simulink model "MdXX_RspChk"  (R2018b)
settings: Solver=FixedStepDiscrete  StartTime=0.0  StopTime=10.0  FixedStep=0.01  RelTol=1e-3
libraries: OutRspChkLib x20
(part 2 of 2)

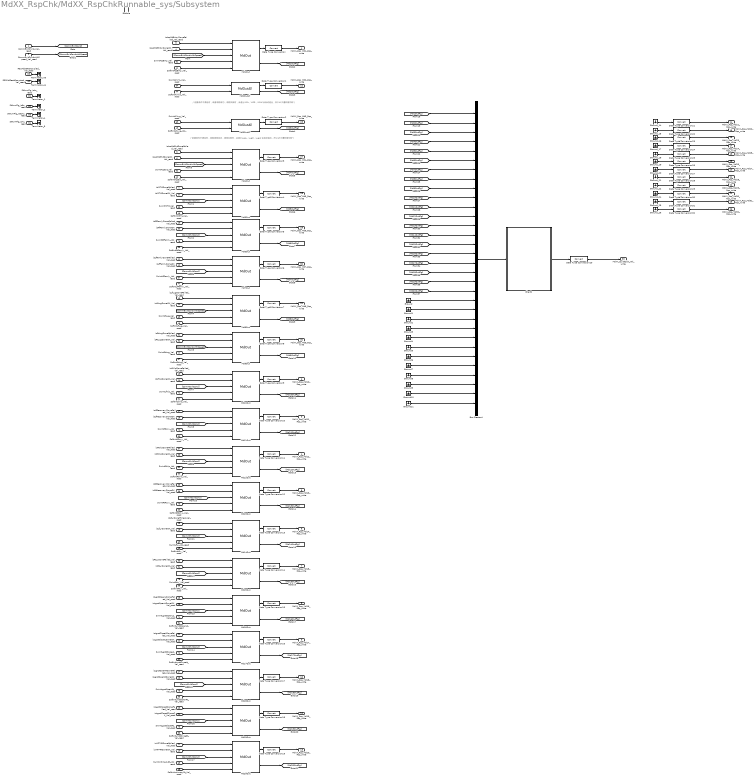
== system MdXX_RspChk/MdXX_RspChkRunnable_sys/Subsystem ==
  note: /*前提条件不满足时，或者调用成功，调用失败时，会退出LugL，LugR，LugAll会自动退出，所以All只看软硬中断*/
  note: /*前提条件不满足时，或者调用成功，调用失败时，会退出VIPL，VIPR，VIPAll会自动退出，所以All只看软硬中断*/
  CommExitCond_Val_read : Inport
  CommExitCondwithSpeed_Val_read : Inport  Port=2
  isAcsMdEntryDoneFailed_Val_read : Inport  Port=3
  isAcsMdEntryDoneOK_Val_read : Inport  Port=4
  isAcsMdExtDoneFailed_Val_read : Inport  Port=5
  isAcsMdExtDoneOK_Val_read : Inport  Port=6
  isINTMDoneFailed_Val_read : Inport  Port=7
  isINTMDoneOK_Val_read : Inport  Port=8
  isINTMRDoneFailed_Val_read : Inport  Port=9
  isINTMRDoneOK_Val_read : Inport  Port=10
  isLfFamlyDoneFailed_Val_read : Inport  Port=11
  isLfFamlyDoneOK_Val_read : Inport  Port=12
  isLfLugDoneFailed_Val_read : Inport  Port=13
  isLfLugDoneOK_Val_read : Inport  Port=14
  isLfLyDoneFailed_Val_read : Inport  Port=15
  isLfLyDoneOK_Val_read : Inport  Port=16
  isLfRecoveryDoneFailed_Val_read : Inport  Port=17
  isLfRecoveryDoneOK_Val_read : Inport  Port=18
  isLfVipDoneFailed_Val_read : Inport  Port=19
  isLfVipDoneOK_Val_read : Inport  Port=20
  isLgrstCloseLDoneFailed_Val_read : Inport  Port=21
  isLgrstCloseLDoneOK_Val_read : Inport  Port=22
  isLgrstCloseRDoneFailed_Val_read : Inport  Port=23
  isLgrstCloseRDoneOK_Val_read : Inport  Port=24
  isLgrstOpenLDoneFailed_Val_read : Inport  Port=25
  isLgrstOpenLDoneOK_Val_read : Inport  Port=26
  isLgrstOpenRDoneFailed_Val_read : Inport  Port=27
  isLgrstOpenRDoneOK_Val_read : Inport  Port=28
  isRfFamlyDoneFailed_Val_read : Inport  Port=29
  isRfFamlyDoneOK_Val_read : Inport  Port=30
  isRtLugDoneFailed_Val_read : Inport  Port=31
  isRtLugDoneOK_Val_read : Inport  Port=32
  isRtLyDoneFailed_Val_read : Inport  Port=33
  isRtLyDoneOK_Val_read : Inport  Port=34
  isRtRecoveryDoneFailed_Val_read : Inport  Port=35
  isRtRecoveryDoneOK_Val_read : Inport  Port=36
  isRtVipDoneFailed_Val_read : Inport  Port=37
  isRtVipDoneOK_Val_read : Inport  Port=38
  R3LMdSeatOccupied_Val_read : Inport  Port=39
  R3RMdSeatOccupied_Val_read : Inport  Port=40
  SoftIntAcsEnty_Val_read : Inport  Port=41
  SoftIntAcsExt_Val_read : Inport  Port=42
  SoftIntAllLug_Val_read : Inport  Port=43
  SoftIntAllVip_Val_read : Inport  Port=44
  SoftIntIntimacyRt_Val_read : Inport  Port=45
  SoftIntINTM_Val_read : Inport  Port=46
  SoftIntLfFamly_Val_read : Inport  Port=47
  SoftIntLfLug_Val_read : Inport  Port=48
  SoftIntLfLy_Val_read : Inport  Port=49
  SoftIntLfRcvy_Val_read : Inport  Port=50
  SoftIntLfVip_Val_read : Inport  Port=51
  SoftIntLgrstCloseLt_Val_read : Inport  Port=52
  SoftIntLgrstCloseRt_Val_read : Inport  Port=53
  SoftIntLgrstOpenLt_Val_read : Inport  Port=54
  SoftIntLgrstOpenRt_Val_read : Inport  Port=55
  SoftIntRtFamly_Val_read : Inport  Port=56
  SoftIntRtLug_Val_read : Inport  Port=57
  SoftIntRtLy_Val_read : Inport  Port=58
  SoftIntRtRcvy_Val_read : Inport  Port=59
  SoftIntRtVip_Val_read : Inport  Port=60
  SwIntAcsEnty_Val_read : Inport  Port=61
  SwIntAcsExt_Val_read : Inport  Port=62
  SwIntAllLug_Val_read : Inport  Port=63
  SwIntAllVip_Val_read : Inport  Port=64
  SwIntIntimacyRt_Val_read : Inport  Port=65
  SwIntINTM_Val_read : Inport  Port=66
  SwIntLfFamly_Val_read : Inport  Port=67
  SwIntLfLug_Val_read : Inport  Port=68
  SwIntLfLy_Val_read : Inport  Port=69
  SwIntLfRcvy_Val_read : Inport  Port=70
  SwIntLfVip_Val_read : Inport  Port=71
  SwIntLgrstCloseLt_Val_read : Inport  Port=72
  SwIntLgrstCloseRt_Val_read : Inport  Port=73
  SwIntLgrstOpenLt_Val_read : Inport  Port=74
  SwIntLgrstOpenRt_Val_read : Inport  Port=75
  SwIntRtFamly_Val_read : Inport  Port=76
  SwIntRtLug_Val_read : Inport  Port=77
  SwIntRtLy_Val_read : Inport  Port=78
  SwIntRtRcvy_Val_read : Inport  Port=79
  SwIntRtVip_Val_read : Inport  Port=80
  StNumFlg_Is4s_read : Inport  Port=81
  StNumFlg_Is6s_read : Inport  Port=82
  StNumFlg_Is6s7s_read : Inport  Port=83
  StNumFlg_Is7s_read : Inport  Port=84
  Enable : EnablePort
  Bus Creator4 : BusCreator  Inputs=32
  Chart2 : Stateflow chart  TreatAsAtomicUnit=on
  Data Type Conversion{,1..32} (33 alike) : DataTypeConversion
  Ground{,1..11} (12 alike) : Ground
  Ground_{14..22,24..26} (12 alike) : Ground
  Md10Out : OutRspChkLib/MdOut  SystemSampleTime=-1
  Md11Out : OutRspChkLib/MdOut  SystemSampleTime=-1
  Md12Out : OutRspChkLib/MdOut  SystemSampleTime=-1
  Md13Out : OutRspChkLib/MdOut  SystemSampleTime=-1
  Md14Out : OutRspChkLib/MdOut  SystemSampleTime=-1
  Md15Out : OutRspChkLib/MdOut  SystemSampleTime=-1
  Md16Out : OutRspChkLib/MdOut  SystemSampleTime=-1
  Md17Out : OutRspChkLib/MdOut  SystemSampleTime=-1
  Md18Out : OutRspChkLib/MdOut  SystemSampleTime=-1
  Md19Out : OutRspChkLib/MdOut  SystemSampleTime=-1
  Md1Out : OutRspChkLib/MdOut  SystemSampleTime=-1
  Md20Out : OutRspChkLib/MdOut  SystemSampleTime=-1
  Md2OutAll : OutRspChkLib/MdOutAll  SystemSampleTime=-1
  Md3OutAll : OutRspChkLib/MdOutAll  SystemSampleTime=-1
  Md4Out : OutRspChkLib/MdOut  SystemSampleTime=-1
  Md5Out : OutRspChkLib/MdOut  SystemSampleTime=-1
  Md6Out : OutRspChkLib/MdOut  SystemSampleTime=-1
  Md7Out : OutRspChkLib/MdOut  SystemSampleTime=-1
  Md8Out : OutRspChkLib/MdOut  SystemSampleTime=-1
  Md9Out : OutRspChkLib/MdOut  SystemSampleTime=-1
  Terminator_{1..2,4..5,43..44} (6 alike) : Terminator
  MdXX_Rsp_Md1_Rsp_write : Outport
  MdXX_Rsp_Md10_Rsp_write : Outport  Port=2
  MdXX_Rsp_Md11_Rsp_write : Outport  Port=3
  MdXX_Rsp_Md12_Rsp_write : Outport  Port=4
  MdXX_Rsp_Md13_Rsp_write : Outport  Port=5
  MdXX_Rsp_Md14_Rsp_write : Outport  Port=6
  MdXX_Rsp_Md15_Rsp_write : Outport  Port=7
  MdXX_Rsp_Md16_Rsp_write : Outport  Port=8
  MdXX_Rsp_Md17_Rsp_write : Outport  Port=9
  MdXX_Rsp_Md18_Rsp_write : Outport  Port=10
  MdXX_Rsp_Md19_Rsp_write : Outport  Port=11
  MdXX_Rsp_Md2_Rsp_write : Outport  Port=12
  MdXX_Rsp_Md20_Rsp_write : Outport  Port=13
  MdXX_Rsp_Md21_Rsp_write : Outport  Port=14
  MdXX_Rsp_Md22_Rsp_write : Outport  Port=15
  MdXX_Rsp_Md23_Rsp_write : Outport  Port=16
  MdXX_Rsp_Md24_Rsp_write : Outport  Port=17
  MdXX_Rsp_Md25_Rsp_write : Outport  Port=18
  MdXX_Rsp_Md26_Rsp_write : Outport  Port=19
  MdXX_Rsp_Md27_Rsp_write : Outport  Port=20
  MdXX_Rsp_Md28_Rsp_write : Outport  Port=21
  MdXX_Rsp_Md29_Rsp_write : Outport  Port=22
  MdXX_Rsp_Md3_Rsp_write : Outport  Port=23
  MdXX_Rsp_Md30_Rsp_write : Outport  Port=24
  MdXX_Rsp_Md31_Rsp_write : Outport  Port=25
  MdXX_Rsp_Md32_Rsp_write : Outport  Port=26
  MdXX_Rsp_Md4_Rsp_write : Outport  Port=27
  MdXX_Rsp_Md5_Rsp_write : Outport  Port=28
  MdXX_Rsp_Md6_Rsp_write : Outport  Port=29
  MdXX_Rsp_Md7_Rsp_write : Outport  Port=30
  MdXX_Rsp_Md8_Rsp_write : Outport  Port=31
  MdXX_Rsp_Md9_Rsp_write : Outport  Port=32
  MdXX_Quit32bit_Val_write : Outport  Port=33
  wires:
  isLfVipDoneFailed_Val_read/1 -> Md10Out/1
  Md1Out/1 -> Data Type Conversion/1
  Ground_18/1 -> Data Type Conversion25/1
  isLgrstOpenLDoneFailed_Val_read/1 -> Md16Out/1
  R3LMdSeatOccupied_Val_read/1 -> Terminator_43/1
  Ground_14/1 -> Data Type Conversion21/1
  SoftIntLgrstCloseRt_Val_read/1 -> Md19Out/5
  SwIntIntimacyRt_Val_read/1 -> Md20Out/4
  isLfFamlyDoneFailed_Val_read/1 -> Md7Out/1
  Ground_19/1 -> Data Type Conversion26/1
  Ground_24/1 -> Data Type Conversion30/1
  isRtVipDoneFailed_Val_read/1 -> Md12Out/1
  Ground_17/1 -> Data Type Conversion24/1
  Ground_20/1 -> Data Type Conversion27/1
  Ground_21/1 -> Data Type Conversion28/1
  isINTMDoneOK_Val_read/1 -> Md5Out/2
  isRfFamlyDoneOK_Val_read/1 -> Md6Out/2
  isLfLugDoneFailed_Val_read/1 -> Md8Out/1
  R3RMdSeatOccupied_Val_read/1 -> Terminator_44/1
  Ground_26/1 -> Data Type Conversion32/1
  isLgrstOpenLDoneOK_Val_read/1 -> Md16Out/2
  Ground_25/1 -> Data Type Conversion31/1
  isRtLugDoneOK_Val_read/1 -> Md9Out/2
  isRtLyDoneOK_Val_read/1 -> Md15Out/2
  isLfFamlyDoneOK_Val_read/1 -> Md7Out/2
  isLgrstOpenRDoneFailed_Val_read/1 -> Md18Out/1
  SoftIntLgrstOpenRt_Val_read/1 -> Md18Out/5
  isLfVipDoneOK_Val_read/1 -> Md10Out/2
  isRtVipDoneOK_Val_read/1 -> Md12Out/2
  CommExitCond_Val_read/1 -> [CommExitCond]
  isRtLyDoneFailed_Val_read/1 -> Md15Out/1
  isRfFamlyDoneFailed_Val_read/1 -> Md6Out/1
  isINTMDoneFailed_Val_read/1 -> Md5Out/1
  Ground_22/1 -> Data Type Conversion29/1
  isLgrstOpenRDoneOK_Val_read/1 -> Md18Out/2
  isINTMRDoneFailed_Val_read/1 -> Md20Out/1
  Ground_16/1 -> Data Type Conversion23/1
  Ground_15/1 -> Data Type Conversion22/1
  CommExitCondwithSpeed_Val_read/1 -> [CommExitCondwithSpeed]
  isLfRecoveryDoneOK_Val_read/1 -> Md11Out/2
  isLfRecoveryDoneFailed_Val_read/1 -> Md11Out/1
  isINTMRDoneOK_Val_read/1 -> Md20Out/2
  isLfLugDoneOK_Val_read/1 -> Md8Out/2
  isRtLugDoneFailed_Val_read/1 -> Md9Out/1
  SwIntAcsEnty_Val_read/1 -> Md1Out/4
  SoftIntAcsEnty_Val_read/1 -> Md1Out/5
  [CommExitCondwithSpeed] -> Md1Out/3
  isAcsMdEntryDoneFailed_Val_read/1 -> Md1Out/1
  isAcsMdEntryDoneOK_Val_read/1 -> Md1Out/2
  Md1Out/2 -> [Md1OutFlg]
  Md3OutAll/1 -> Data Type Conversion2/1
  Md2OutAll/1 -> Data Type Conversion1/1
  Md4Out/1 -> Data Type Conversion3/1
  Md5Out/1 -> Data Type Conversion4/1
  Md6Out/1 -> Data Type Conversion5/1
  Md7Out/1 -> Data Type Conversion6/1
  Md8Out/1 -> Data Type Conversion7/1
  Md9Out/1 -> Data Type Conversion8/1
  Md10Out/1 -> Data Type Conversion9/1
  Md11Out/1 -> Data Type Conversion10/1
  Md12Out/1 -> Data Type Conversion11/1
  Md13Out/1 -> Data Type Conversion12/1
  Md14Out/1 -> Data Type Conversion13/1
  Md15Out/1 -> Data Type Conversion14/1
  Md16Out/1 -> Data Type Conversion15/1
  Md17Out/1 -> Data Type Conversion16/1
  Md18Out/1 -> Data Type Conversion17/1
  Md19Out/1 -> Data Type Conversion18/1
  Md20Out/1 -> Data Type Conversion19/1
  Md2OutAll/2 -> [Md2OutFlg]
  Md3OutAll/2 -> [Md3OutFlg]
  Md4Out/2 -> [Md4OutFlg]
  Md5Out/2 -> [Md5OutFlg]
  Md6Out/2 -> [Md6OutFlg]
  Md7Out/2 -> [Md7OutFlg]
  Md8Out/2 -> [Md8OutFlg]
  Md9Out/2 -> [Md9OutFlg]
  Md10Out/2 -> [Md10OutFlg]
  Md11Out/2 -> [Md11OutFlg]
  Md12Out/2 -> [Md12OutFlg]
  Md13Out/2 -> [Md13OutFlg]
  Md14Out/2 -> [Md14OutFlg]
  Md15Out/2 -> [Md15OutFlg]
  Md16Out/2 -> [Md16OutFlg]
  Md17Out/2 -> [Md17OutFlg]
  Md18Out/2 -> [Md18OutFlg]
  Md19Out/2 -> [Md19OutFlg]
  Md20Out/2 -> [Md20OutFlg]
  isAcsMdExtDoneFailed_Val_read/1 -> Md4Out/1
  isAcsMdExtDoneOK_Val_read/1 -> Md4Out/2
  isRtRecoveryDoneFailed_Val_read/1 -> Md13Out/1
  isRtRecoveryDoneOK_Val_read/1 -> Md13Out/2
  isLfLyDoneFailed_Val_read/1 -> Md14Out/1
  isLfLyDoneOK_Val_read/1 -> Md14Out/2
  isLgrstCloseLDoneFailed_Val_read/1 -> Md17Out/1
  isLgrstCloseLDoneOK_Val_read/1 -> Md17Out/2
  isLgrstCloseRDoneFailed_Val_read/1 -> Md19Out/1
  isLgrstCloseRDoneOK_Val_read/1 -> Md19Out/2
  [CommExitCondwithSpeed] -> Md4Out/3
  [CommExitCondwithSpeed] -> Md8Out/3
  [CommExitCondwithSpeed] -> Md9Out/3
  [CommExitCond] -> Md5Out/3
  [CommExitCond] -> Md6Out/3
  [CommExitCond] -> Md7Out/3
  [CommExitCond] -> Md10Out/3
  [CommExitCond] -> Md11Out/3
  [CommExitCond] -> Md12Out/3
  [CommExitCond] -> Md13Out/3
  [CommExitCond] -> Md14Out/3
  [CommExitCond] -> Md15Out/3
  [CommExitCond] -> Md16Out/3
  [CommExitCond] -> Md17Out/3
  [CommExitCond] -> Md18Out/3
  [CommExitCond] -> Md19Out/3
  [CommExitCond] -> Md20Out/3
  SwIntLgrstCloseRt_Val_read/1 -> Md19Out/4
  SwIntLgrstOpenRt_Val_read/1 -> Md18Out/4
  SwIntLgrstOpenLt_Val_read/1 -> Md16Out/4
  SwIntLgrstCloseLt_Val_read/1 -> Md17Out/4
  SwIntRtLy_Val_read/1 -> Md15Out/4
  SwIntLfLy_Val_read/1 -> Md14Out/4
  SwIntRtRcvy_Val_read/1 -> Md13Out/4
  SwIntRtVip_Val_read/1 -> Md12Out/4
  SwIntLfRcvy_Val_read/1 -> Md11Out/4
  SwIntLfVip_Val_read/1 -> Md10Out/4
  SwIntLfLug_Val_read/1 -> Md8Out/4
  SwIntLfFamly_Val_read/1 -> Md7Out/4
  SwIntRtFamly_Val_read/1 -> Md6Out/4
  SwIntINTM_Val_read/1 -> Md5Out/4
  SoftIntAllLug_Val_read/1 -> Md3OutAll/2
  SoftIntAllVip_Val_read/1 -> Md2OutAll/2
  SoftIntINTM_Val_read/1 -> Md5Out/5
  SoftIntAcsExt_Val_read/1 -> Md4Out/5
  SwIntAllLug_Val_read/1 -> Md3OutAll/1
  SwIntAllVip_Val_read/1 -> Md2OutAll/1
  SwIntAcsExt_Val_read/1 -> Md4Out/4
  SoftIntLfFamly_Val_read/1 -> Md7Out/5
  SoftIntRtFamly_Val_read/1 -> Md6Out/5
  SwIntRtLug_Val_read/1 -> Md9Out/4
  SoftIntLfVip_Val_read/1 -> Md10Out/5
  SoftIntLfRcvy_Val_read/1 -> Md11Out/5
  SoftIntRtVip_Val_read/1 -> Md12Out/5
  SoftIntRtRcvy_Val_read/1 -> Md13Out/5
  SoftIntLfLy_Val_read/1 -> Md14Out/5
  SoftIntRtLy_Val_read/1 -> Md15Out/5
  SoftIntLgrstCloseLt_Val_read/1 -> Md17Out/5
  SoftIntRtLug_Val_read/1 -> Md9Out/5
  SoftIntLfLug_Val_read/1 -> Md8Out/5
  SoftIntIntimacyRt_Val_read/1 -> Md20Out/5
  Chart2/1(Data32Bit) -> Data Type Conversion20/1
  Bus Creator4/1 -> Chart2/1(DataArray)  "MdQuitFlg"
  [Md1OutFlg] -> Bus Creator4/1
  [Md2OutFlg] -> Bus Creator4/2
  [Md3OutFlg] -> Bus Creator4/3
  [Md4OutFlg] -> Bus Creator4/4
  [Md5OutFlg] -> Bus Creator4/5
  [Md6OutFlg] -> Bus Creator4/6
  [Md7OutFlg] -> Bus Creator4/7
  [Md8OutFlg] -> Bus Creator4/8
  [Md9OutFlg] -> Bus Creator4/9
  [Md10OutFlg] -> Bus Creator4/10
  [Md11OutFlg] -> Bus Creator4/11
  [Md12OutFlg] -> Bus Creator4/12
  [Md13OutFlg] -> Bus Creator4/13
  [Md14OutFlg] -> Bus Creator4/14
  [Md15OutFlg] -> Bus Creator4/15
  [Md16OutFlg] -> Bus Creator4/16
  [Md17OutFlg] -> Bus Creator4/17
  [Md18OutFlg] -> Bus Creator4/18
  [Md19OutFlg] -> Bus Creator4/19
  [Md20OutFlg] -> Bus Creator4/20
  Ground/1 -> Bus Creator4/21
  Ground1/1 -> Bus Creator4/22
  Ground2/1 -> Bus Creator4/23
  Ground3/1 -> Bus Creator4/24
  Ground4/1 -> Bus Creator4/25
  Ground5/1 -> Bus Creator4/26
  Ground6/1 -> Bus Creator4/27
  Ground7/1 -> Bus Creator4/28
  Ground8/1 -> Bus Creator4/29
  Ground9/1 -> Bus Creator4/30
  Ground10/1 -> Bus Creator4/31
  Ground11/1 -> Bus Creator4/32
  Data Type Conversion/1 -> MdXX_Rsp_Md1_Rsp_write/1
  Data Type Conversion1/1 -> MdXX_Rsp_Md2_Rsp_write/1
  Data Type Conversion2/1 -> MdXX_Rsp_Md3_Rsp_write/1
  Data Type Conversion3/1 -> MdXX_Rsp_Md4_Rsp_write/1
  Data Type Conversion4/1 -> MdXX_Rsp_Md5_Rsp_write/1
  Data Type Conversion5/1 -> MdXX_Rsp_Md6_Rsp_write/1
  Data Type Conversion6/1 -> MdXX_Rsp_Md7_Rsp_write/1
  Data Type Conversion7/1 -> MdXX_Rsp_Md8_Rsp_write/1
  Data Type Conversion8/1 -> MdXX_Rsp_Md9_Rsp_write/1
  Data Type Conversion9/1 -> MdXX_Rsp_Md10_Rsp_write/1
  Data Type Conversion10/1 -> MdXX_Rsp_Md11_Rsp_write/1
  Data Type Conversion11/1 -> MdXX_Rsp_Md12_Rsp_write/1
  Data Type Conversion12/1 -> MdXX_Rsp_Md13_Rsp_write/1
  Data Type Conversion13/1 -> MdXX_Rsp_Md14_Rsp_write/1
  Data Type Conversion14/1 -> MdXX_Rsp_Md15_Rsp_write/1
  Data Type Conversion15/1 -> MdXX_Rsp_Md16_Rsp_write/1
  Data Type Conversion16/1 -> MdXX_Rsp_Md17_Rsp_write/1
  Data Type Conversion17/1 -> MdXX_Rsp_Md18_Rsp_write/1
  Data Type Conversion18/1 -> MdXX_Rsp_Md19_Rsp_write/1
  Data Type Conversion19/1 -> MdXX_Rsp_Md20_Rsp_write/1
  Data Type Conversion20/1 -> MdXX_Quit32bit_Val_write/1
  SoftIntLgrstOpenLt_Val_read/1 -> Md16Out/5
  StNumFlg_Is4s_read/1 -> Terminator_1/1
  StNumFlg_Is6s_read/1 -> Terminator_2/1
  StNumFlg_Is6s7s_read/1 -> Terminator_4/1
  StNumFlg_Is7s_read/1 -> Terminator_5/1
  Data Type Conversion21/1 -> MdXX_Rsp_Md21_Rsp_write/1
  Data Type Conversion22/1 -> MdXX_Rsp_Md22_Rsp_write/1
  Data Type Conversion23/1 -> MdXX_Rsp_Md23_Rsp_write/1
  Data Type Conversion24/1 -> MdXX_Rsp_Md24_Rsp_write/1
  Data Type Conversion25/1 -> MdXX_Rsp_Md25_Rsp_write/1
  Data Type Conversion26/1 -> MdXX_Rsp_Md26_Rsp_write/1
  Data Type Conversion27/1 -> MdXX_Rsp_Md27_Rsp_write/1
  Data Type Conversion28/1 -> MdXX_Rsp_Md28_Rsp_write/1
  Data Type Conversion29/1 -> MdXX_Rsp_Md29_Rsp_write/1
  Data Type Conversion30/1 -> MdXX_Rsp_Md30_Rsp_write/1
  Data Type Conversion31/1 -> MdXX_Rsp_Md31_Rsp_write/1
  Data Type Conversion32/1 -> MdXX_Rsp_Md32_Rsp_write/1

== stateflow chart MdXX_RspChk/MdXX_RspChkRunnable_sys/Subsystem/Chart2 ==
  (default) -> (junction 3) : {Data32Bit = 0x00000000;}
  (junction 3) -> (junction 9) : {i = 0;}
  (junction 9) -> (junction 4) [order 1] : [i < 32]
  (junction 4) -> (junction 1) : {
      | temp_var = uint32(DataArray[i]);
      | temp_var= temp_var << i;
      | Data32Bit = Data32Bit |  temp_var;
      | }
  (junction 1) -> (junction 9) : {i++;}
  (junction 9) -> (junction 5) [order 2]
  data: Data32Bit output uint32; DataArray input boolean size=32; temp_var local uint32; i local uint8
